simulink model "sampleModel1635"  (R2023a)
settings: Solver=VariableStepAuto  StartTime=0.0  StopTime=10.0  RelTol=1e-3
libraries: hdlsllib x5, simulink x2
settings Model: Creator=user1  LastModifiedBy=user1

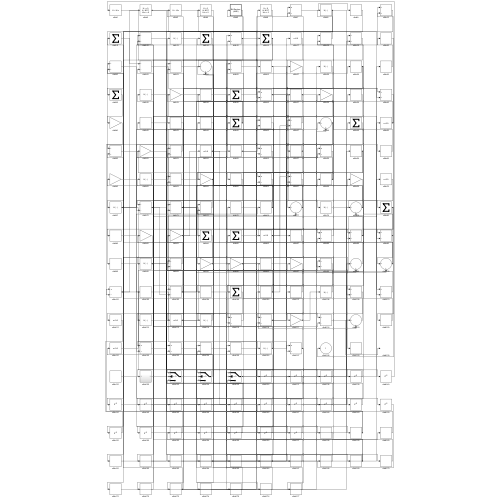
[thumbnail: Simulink's stored preview of the top-level diagram]
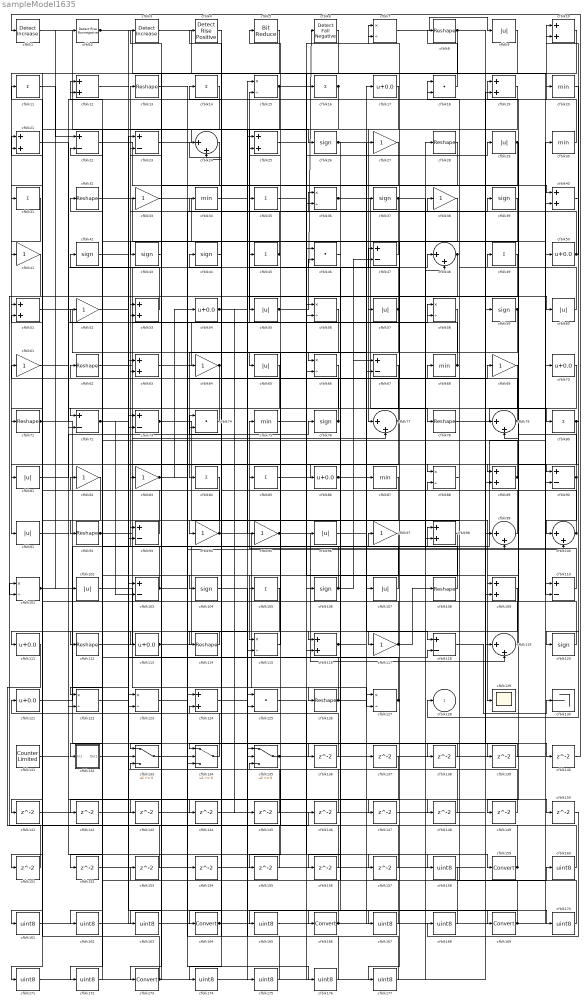
== system sampleModel1635 ==
  cfblk1 : simulink/Logic and Bit Operations/Detect Increase  vinit=0.0  OutDataTypeStr=boolean
      settings: LibrarySourceBlock=|
      | hdlsllib/Logic and Bit
      | Operations/Detect
      | Increase
  cfblk{10,12,19,21,25,40,51,53,63,89,98,109,116,124} (14 alike) : Sum
  cfblk{24,48,77,79,99..100,119} (7 alike) : Sum  Inputs=|++
  cfblk{7,15,36,56,58,66,88,101,115,122..123,127} (12 alike) : Product  Inputs=*/  RndMeth=Zero  SaturateOnIntegerOverflow=on
  cfblk{9,29,55,57,60,65,81,91,96,102,107} (11 alike) : Abs  SaturateOnIntegerOverflow=off
  cfblk{22..23,47,67,72..73,90,93,103,110,118} (11 alike) : Sum  Inputs=+-
  cfblk{26,37,39,42..44,59,76,104,106,120} (11 alike) : Signum
  cfblk{11,14,16,31,35,45,49,80,84..85,105} (11 alike) : Sum  Inputs=+
  cfblk{8,13,28,32,62,71,78,92,108,112,114,126} (12 alike) : Reshape
  cfblk{17,50,54,70,86,111,113,121} (8 alike) : Bias  Bias=0.0  SaturateOnIntegerOverflow=off
  cfblk{27,33,38,41,52,61,64,69,82..83,94..95,97,117} (14 alike) : Gain
  cfblk{18,46,74,125} (4 alike) : DotProduct  OutDataTypeStr=Inherit: Inherit via internal rule
  cfblk129 : Scope
  cfblk130 : Terminator
  cfblk131 : hdlsllib/Sources/Counter Limited  uplimit=7  tsamp=-1
  cfblk132 : Subsystem
      settings: LibrarySourceBlock=|
      | hdlsllib/Ports &
      | Subsystems/Subsystem
  cfblk133 : Switch  SaturateOnIntegerOverflow=off  InputSameDT=off
  cfblk134 : Switch  SaturateOnIntegerOverflow=off  InputSameDT=off
  cfblk135 : Switch  SaturateOnIntegerOverflow=off  InputSameDT=off
  cfblk{136..157} (22 alike) : Delay  SampleTime=1
  cfblk{158,160..163,165,167..168,170..172,174..177} (15 alike) : DataTypeConversion  OutDataTypeStr=uint8  SaturateOnIntegerOverflow=off  RndMeth=Floor
  cfblk{159,164,166,169,173} (5 alike) : DataTypeConversion  SaturateOnIntegerOverflow=off  RndMeth=Floor
  cfblk2 : hdlsllib/Logic and Bit Operations/Detect Rise Nonnegative  vinit=0  OutDataTypeStr=boolean
  cfblk{20,30,34,68,75,87} (6 alike) : MinMax
  cfblk3 : simulink/Logic and Bit Operations/Detect Increase  vinit=0.0  OutDataTypeStr=boolean
      settings: LibrarySourceBlock=|
      | hdlsllib/Logic and Bit
      | Operations/Detect
      | Increase
  cfblk4 : hdlsllib/Logic and Bit Operations/Detect Rise Positive  vinit=0  OutDataTypeStr=boolean
  cfblk5 : hdlsllib/Logic and Bit Operations/Bit Reduce  mode=AND
  cfblk6 : hdlsllib/Logic and Bit Operations/Detect Fall Negative  vinit=0  OutDataTypeStr=boolean
  cfblk128 : Outport  VectorParamsAs1DForOutWhenUnconnected=off
  wires:
  cfblk9/1 -> cfblk91/1
  cfblk83/1 -> cfblk54/1, cfblk39/1
  cfblk99/1 -> cfblk14/1
  cfblk17/1 -> cfblk77/1
  cfblk77/1 -> cfblk3/1, cfblk24/1, cfblk141/1
  cfblk108/1 -> cfblk13/1
  cfblk70/1 -> cfblk94/1
  cfblk30/1 -> cfblk10/1
  cfblk36/1 -> cfblk78/1, cfblk98/2
  cfblk126/1 -> cfblk62/1, cfblk58/2
  cfblk11/1 -> cfblk22/1
  cfblk16/1 -> cfblk143/1, cfblk144/1
  cfblk113/1 -> cfblk17/1, cfblk150/1
  cfblk114/1 -> cfblk111/1
  cfblk122/1 -> cfblk97/1
  cfblk62/1 -> cfblk58/1
  cfblk74/1 -> cfblk72/1
  cfblk66/1 -> cfblk104/1
  cfblk63/1 -> cfblk15/2
  cfblk94/1 -> cfblk126/1, cfblk12/2
  cfblk73/1 -> cfblk129/1, cfblk99/2, cfblk115/2
  cfblk15/1 -> cfblk55/1, cfblk7/1
  cfblk71/1 -> cfblk123/2, cfblk48/1, cfblk53/2
  cfblk117/1 -> cfblk5/1, cfblk108/1
  cfblk78/1 -> cfblk80/1
  cfblk98/1 -> cfblk115/1
  cfblk92/1 -> cfblk77/2, cfblk157/1
  cfblk55/1 -> cfblk6/1, cfblk90/2
  cfblk47/1 -> cfblk43/1
  cfblk120/1 -> cfblk79/2
  cfblk56/1 -> cfblk84/1
  cfblk69/1 -> cfblk117/1
  cfblk24/1 -> cfblk133/1
  cfblk96/1 -> cfblk37/1
  cfblk23/1 -> cfblk26/1
  cfblk119/1 -> cfblk21/1
  cfblk38/1 -> cfblk92/1
  cfblk134/1 -> cfblk121/1
  cfblk121/1 -> cfblk50/1
  cfblk118/1 -> cfblk130/1
  cfblk45/1 -> cfblk35/1, cfblk24/2
  cfblk127/1 -> cfblk42/1, cfblk177/1
  cfblk110/1 -> cfblk75/1
  cfblk112/1 -> cfblk47/1
  cfblk79/1 -> cfblk44/1, cfblk7/2
  cfblk51/1 -> cfblk87/1
  cfblk31/1 -> cfblk41/1
  cfblk10/1 -> cfblk71/1
  cfblk68/1 -> cfblk18/1, cfblk66/1, cfblk53/1
  cfblk34/1 -> cfblk60/1
  cfblk116/1 -> cfblk107/1, cfblk98/1
  cfblk86/1 -> cfblk118/1, cfblk67/1
  cfblk40/1 -> cfblk128/1
  cfblk125/1 -> cfblk159/1
  cfblk89/1 -> cfblk32/1, cfblk19/1
  cfblk58/1 -> cfblk65/1
  cfblk29/1 -> cfblk109/1, cfblk67/2, cfblk156/1
  cfblk72/1 -> cfblk103/2, cfblk138/1
  cfblk57/1 -> cfblk45/1, cfblk155/1
  cfblk25/1 -> cfblk56/1
  cfblk4/1 -> cfblk64/1
  cfblk85/1 -> cfblk89/1
  cfblk28/1 -> cfblk173/1
  cfblk133/1 -> cfblk36/1
  cfblk101/1 -> cfblk134/3, cfblk2/1
  cfblk132/1(Out1) -> cfblk118/2
  cfblk135/1 -> cfblk59/1, cfblk30/1
  cfblk7/1 -> cfblk9/1
  cfblk84/1 -> cfblk112/1
  cfblk90/1 -> cfblk100/1, cfblk49/1
  cfblk1/1 -> cfblk95/1
  cfblk88/1 -> cfblk38/1
  cfblk48/1 -> cfblk81/1, cfblk57/1
  cfblk20/1 -> cfblk90/1
  cfblk18/1 -> cfblk8/1
  cfblk32/1 -> cfblk86/1
  cfblk54/1 -> cfblk89/2, cfblk145/1
  cfblk67/1 -> cfblk105/1
  cfblk27/1 -> cfblk164/1
  cfblk5/1 -> cfblk51/1
  cfblk14/1 -> cfblk31/1
  cfblk41/1 -> cfblk101/2
  cfblk42/1 -> cfblk133/2
  cfblk8/1 -> cfblk113/1, cfblk93/2, cfblk140/1
  cfblk100/1 -> cfblk74/1, cfblk85/1
  cfblk106/1 -> cfblk93/1, cfblk47/2
  cfblk61/1 -> cfblk20/1
  cfblk103/1 -> cfblk12/1, cfblk68/1, cfblk69/1
  cfblk95/1 -> cfblk119/2, cfblk96/1
  cfblk53/1 -> cfblk22/2
  cfblk49/1 -> cfblk72/2
  cfblk26/1 -> cfblk40/2, cfblk136/1
  cfblk107/1 -> cfblk63/2
  cfblk33/1 -> cfblk110/1
  cfblk60/1 -> cfblk33/1
  cfblk59/1 -> cfblk116/1, cfblk66/2
  cfblk80/1 -> cfblk120/1, cfblk149/1
  cfblk102/1 -> cfblk127/2
  cfblk46/1 -> cfblk166/1
  cfblk97/1 -> cfblk132/1(In1)
  cfblk3/1 -> cfblk110/2
  cfblk81/1 -> cfblk76/1
  cfblk93/1 -> cfblk51/2
  cfblk22/1 -> cfblk40/1
  cfblk64/1 -> cfblk34/1, cfblk122/2
  cfblk21/1 -> cfblk102/1
  cfblk35/1 -> cfblk29/1
  cfblk50/1 -> cfblk23/2, cfblk10/2
  cfblk76/1 -> cfblk61/1, cfblk4/1
  cfblk2/1 -> cfblk36/2, cfblk88/1
  cfblk115/1 -> cfblk25/2
  cfblk37/1 -> cfblk100/2, cfblk122/1
  cfblk52/1 -> cfblk169/1
  cfblk105/1 -> cfblk114/1
  cfblk75/1 -> cfblk109/2
  cfblk136/1 -> cfblk23/1
  cfblk138/1 -> cfblk134/1
  cfblk12/1 -> cfblk139/1
  cfblk139/1 -> cfblk135/2
  cfblk140/1 -> cfblk1/1
  cfblk141/1 -> cfblk15/1
  cfblk109/1 -> cfblk142/1
  cfblk142/1 -> cfblk99/1
  cfblk144/1 -> cfblk116/2
  cfblk145/1 -> cfblk63/1
  cfblk111/1 -> cfblk146/1
  cfblk146/1 -> cfblk74/2
  cfblk39/1 -> cfblk147/1
  cfblk147/1 -> cfblk79/1
  cfblk91/1 -> cfblk148/1
  cfblk148/1 -> cfblk123/1
  cfblk149/1 -> cfblk133/3
  cfblk87/1 -> cfblk151/1
  cfblk151/1 -> cfblk101/1
  cfblk65/1 -> cfblk152/1
  cfblk152/1 -> cfblk127/1
  cfblk153/1 -> cfblk103/1
  cfblk13/1 -> cfblk154/1
  cfblk154/1 -> cfblk119/1
  cfblk155/1 -> cfblk134/2
  cfblk156/1 -> cfblk21/2
  cfblk157/1 -> cfblk135/3
  cfblk131/1 -> cfblk158/1
  cfblk159/1 -> cfblk88/2, cfblk73/1
  cfblk158/1 -> cfblk160/1
  cfblk160/1 -> cfblk125/1
  cfblk6/1 -> cfblk161/1
  cfblk161/1 -> cfblk125/2
  cfblk137/1 -> cfblk162/1
  cfblk162/1 -> cfblk73/2
  cfblk43/1 -> cfblk163/1
  cfblk163/1 -> cfblk137/1
  cfblk164/1 -> cfblk106/1, cfblk70/1
  cfblk165/1 -> cfblk27/1
  cfblk166/1 -> cfblk48/2, cfblk25/1
  cfblk123/1 -> cfblk167/1
  cfblk167/1 -> cfblk46/1
  cfblk150/1 -> cfblk168/1
  cfblk168/1 -> cfblk46/2
  cfblk169/1 -> cfblk165/1, cfblk153/1, cfblk18/2
  cfblk104/1 -> cfblk170/1
  cfblk170/1 -> cfblk52/1
  cfblk82/1 -> cfblk171/1
  cfblk171/1 -> cfblk56/2
  cfblk19/1 -> cfblk172/1
  cfblk172/1 -> cfblk82/1
  cfblk173/1 -> cfblk19/2, cfblk83/1, cfblk11/1, cfblk16/1
  cfblk44/1 -> cfblk174/1
  cfblk174/1 -> cfblk28/1
  cfblk124/1 -> cfblk175/1
  cfblk175/1 -> cfblk135/1
  cfblk143/1 -> cfblk176/1
  cfblk176/1 -> cfblk124/1
  cfblk177/1 -> cfblk124/2

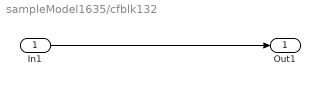
== system sampleModel1635/cfblk132 ==
  In1 : Inport
  Out1 : Outport
  wires:
  In1/1 -> Out1/1
